simulink model "CrazyFlie"  (R2024a)
settings: Solver=FixedStepAuto  StartTime=0.0  StopTime=8  FixedStep=0.002  RelTol=1e-3
model workspace (MAT data in the model file):
  Bias = 0
  Cd = 7.9379e-12
  ControllerType = 1
  Ct = 3.1582e-10
  Ixx = 1.395e-05
  Iyy = 1.436e-05
  Izz = 2.173e-05
  SampleTime = 0.01
  Ts = 100
  d = 0.06761
  density = 5e-06
undefined symbols (not defined in the file): deg, I, I_inv, k_q, k_t, rad, s
libraries: dspindex x14, simulink_extras x11, aerolibconvert2 x7, uavsim3dlib x3, aerolibutil x2, sharedutil x2, sharedtransform x2, matrix_library x1, sim3dlib x1, uavutilslib x1
settings Model: SnapshotInterval=1  Creator=Guy  LastModifiedBy=User
settings OptimizationCC: ReuseModelBlockBuffer=off
settings ModelReferenceCC: EnableRefExpFcnMdlSchedulingChecks=on
settings RTWCC: GPUComputeCapability=3.5

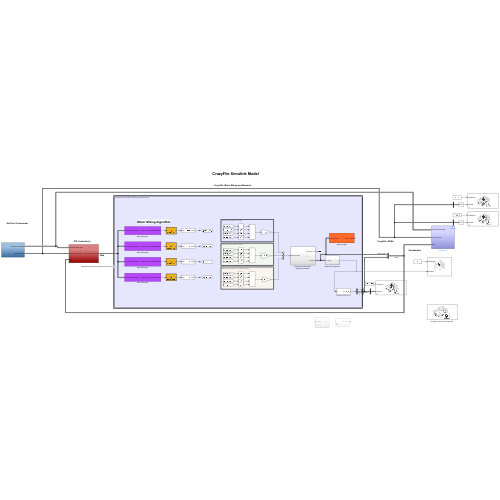
[thumbnail: Simulink's stored preview of the top-level diagram]
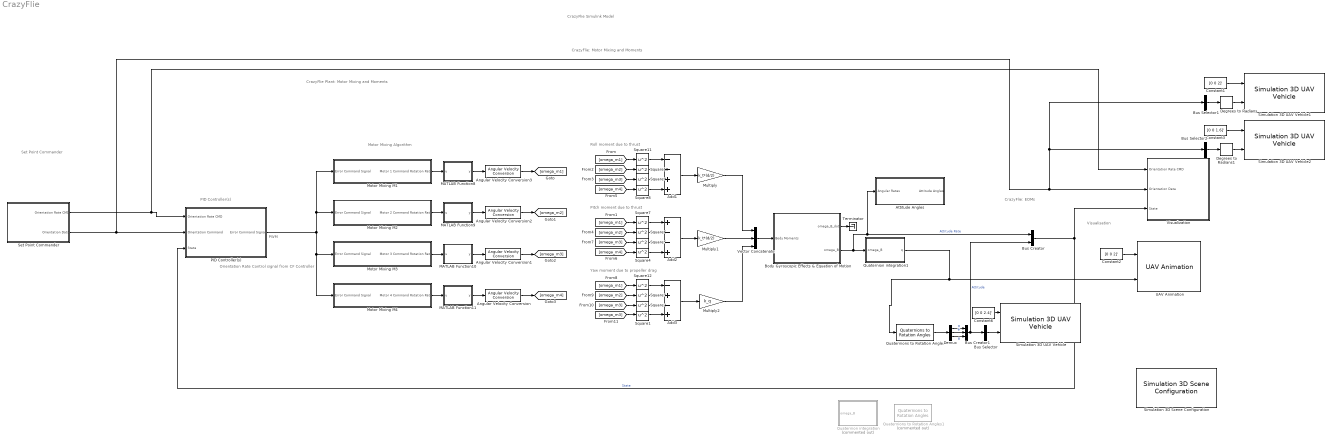
== system CrazyFlie ==
  note: CrazyFlie Plant: Motor Mixing and Moments
  note: PWM
  note: Visualisation
  note: CrazyFlie: EOMs
  note: CrazyFlie: Motor Mixing and Moments
  note: PID Controller(s)
  note: Set Point Commander
  note: CrazyFlie Simulink Model
  note: Orientation Rate Control signal from CF Controller
  note: Motor Mixing Algorithm
  note: Pitch moment due to thrust
  note: Yaw moment due to propeller drag
  note: Roll moment due to thrust
  Add1 : Sum  Inputs=--++
  Add2 : Sum  Inputs=+--+
  Add3 : Sum  Inputs=-+-+
  Angular Velocity Conversion{,1..3} (4 alike) : aerolibconvert2/Angular Velocity Conversion  IU=rpm  OU=rad/s
  Attitude Angles : Subsystem
  Body Gyroscopic Effects & Equation of Motion : Subsystem
  Bus Creator : BusCreator  Inputs=2
  Bus Creator1 : BusCreator  Inputs=3
  Bus Selector : BusSelector  OutputSignals=ψ,Φ,θ  OutputAsBus=on
  Bus Selector1 : BusSelector  OutputSignals=EstimateYaw,EstimatePitch,EstimateRoll  OutputAsBus=on
  Bus Selector2 : BusSelector  OutputSignals=Yaw,Pitch,Roll  OutputAsBus=on
  Constant1 : Constant  Value=[0 0 2]'
  Constant2 : Constant  Value=[0 0 2]'
  Constant3 : Constant  Value=[0 0 1.6]'
  Constant6 : Constant  Value=[0 0 2.4]'
  Degrees to Radians : simulink_extras/Transformations/Degrees to Radians
  Degrees to Radians1 : simulink_extras/Transformations/Degrees to Radians
  Demux : Demux  Outputs=3
  MATLAB Function10 : MATLAB Function  TreatAsAtomicUnit=on
  MATLAB Function11 : MATLAB Function  TreatAsAtomicUnit=on
  MATLAB Function8 : MATLAB Function  TreatAsAtomicUnit=on
  MATLAB Function9 : MATLAB Function  TreatAsAtomicUnit=on
  Motor Mixing M1 : Subsystem
  Motor Mixing M2 : Subsystem
  Motor Mixing M3 : Subsystem
  Motor Mixing M4 : Subsystem
  Multiply : Gain  Gain=k_t*(d/2)
  Multiply1 : Gain  Gain=k_t*(d/2)
  Multiply2 : Gain  Gain=k_q
  PID Controller(s) : Subsystem
  Quaternion integration : Subsystem  Commented=on
  Quaternion integration1 : Subsystem
  Quaternions to Rotation Angles : sharedtransform/Quaternions to Rotation Angles  rotationOrder=ZYX  aMode=aMode
  Quaternions to Rotation Angles1 : sharedtransform/Quaternions to Rotation Angles  Commented=on  rotationOrder=ZYX  aMode=aMode
  Set Point Commander : Subsystem  Tag=Signal Editor
  Simulation 3D Scene Configuration : sim3dlib/Simulation 3D Scene Configuration  Priority=0  ProjectFormat=Default Scenes  SceneDesc=US city block  ProjectName=C:\Program Files\MATLAB\R2024a\toolbox\shared\sim3d_projects\automotive_project_windows\UE\WindowsNoEditor\VehicleSimulation.exe  ScenePath=/Game/Maps/USCityBlock  EnableOpenDRIVE=off  vehTagList={'Custom';'Scene Origin';'SimulinkVehicle1';'SimulinkVehicle2';'SimulinkVehicle3'}  vehTag=Custom  FreeCameraInitialTranslation=[-1.8, 0, 2.6]  FreeCameraDefaultInitialTranslation=[-6, 0, 2]  FreeCameraInitialRotation=[0, -10, 0]  FreeCameraDefaultInitialRotation=[0, -15, 0]  OpVisEn=off  Ts=0.03  EnableWindow=on  EnableRemoteAccess=off  EnableWeather=off  SunAzimuth=90  SunAltitude=40.0  EnableGeospatialSun=off  Latitude=0  Longitude=0  Date=2023-01-01  Time=10:30:00  GeoTimeZone=-5.0  SunDaylightSaving=off  wind=1  clouds=10  EnableVolumetricClouds=off  CloudCoverage=0  CloudAltitude=6  fog=0  rain=0  RaindropsEffect=off  SnowDensity=0  EnableGeospatial=off  UseTrueOrigin=off  OriginHeight=200  OriginLatitude=40.744652  OriginLongitude=-73.988864  MapStyle=Aerial  AdditionalAssetIDs=[]  UseAdvancedSunSky=off  SolarTime=11  TimeZone=-5  Day=21  Month=9  Year=2022  UseDaylightSavingTime=on  DSTStartDay=10  DSTStartMonth=3  DSTEndDay=3  DSTEndMonth=11  DSTSwitchHour=2  sensorTag=MainCamera1  sensorId=1  sensorName=MainCamera1  mountLoc=Origin  offsetFlag=off  tmountOffset=[0, 0, 0]  rmountOffset=[0, 0, 0]  HorizontalResolution=1280  VerticalResolution=720  HorizontalFOV=60  mountPoint=[0 0 0]  mountOrientation=[0 0 0]  aMode=4  ID=1  GeoTrigger=Inactive
      settings: LibrarySourceBlock=uavsim3dlib/Simulation 3D Scene Configuration
  Simulation 3D UAV Vehicle : uavsim3dlib/Simulation 3D UAV Vehicle  Priority=-1  Mesh=Quadrotor  MeshPath=/MathWorksUAVContent/UAVs/HexaRotorUAV/HexaRotor.HexaRotor  Color=Black  ActorName=SimulinkVehicle1  UseGlobalFrame=off  InitialTranslation=[0 0 2.4]  InitialRotation=[0 0 0]  InitialTranslationGlobal=[0 0 0]  InitialGeoOrigin=[0 0 0]  InitialRotationGlobal=[0 0 0]  SampleTime=-1  ActorType=SimulinkVehicle  ID=1  aMode=4  ActorTag=SimulinkVehicle1
  Simulation 3D UAV Vehicle1 : uavsim3dlib/Simulation 3D UAV Vehicle  Priority=-1  Mesh=Quadrotor  MeshPath=/MathWorksUAVContent/UAVs/HexaRotorUAV/HexaRotor.HexaRotor  Color=Black  ActorName=SimulinkVehicle2  UseGlobalFrame=off  InitialTranslation=[0 0 2]  InitialRotation=[0 0 0]  InitialTranslationGlobal=[0 0 0]  InitialGeoOrigin=[0 0 0]  InitialRotationGlobal=[0 0 0]  SampleTime=-1  ActorType=SimulinkVehicle  ID=2  aMode=4  ActorTag=SimulinkVehicle2
  Simulation 3D UAV Vehicle2 : uavsim3dlib/Simulation 3D UAV Vehicle  Priority=-1  Mesh=Quadrotor  MeshPath=/MathWorksUAVContent/UAVs/HexaRotorUAV/HexaRotor.HexaRotor  Color=Black  ActorName=SimulinkVehicle3  UseGlobalFrame=off  InitialTranslation=[0 0 1.6]  InitialRotation=[0 0 0]  InitialTranslationGlobal=[0 0 0]  InitialGeoOrigin=[0 0 0]  InitialRotationGlobal=[0 0 0]  SampleTime=-1  ActorType=SimulinkVehicle  ID=3  aMode=4  ActorTag=SimulinkVehicle3
  Square{1..12} (12 alike) : Math  Operator=square
  Terminator : Terminator
  UAV Animation : uavutilslib/UAV Animation  UAVType=Multirotor  UAVSize=1  InertialZDirection=Up  SampleTime=-1
  Vector Concatenate : Concatenate  NumInputs=3
  Visualization : Subsystem
  wires:
  Set Point Commander/1(Orientation Rate CMD) -> PID Controller(s)/1(Orientation Rate CMD), Visualization/1(Orientation Rate CMD)
  Bus Creator/1 -> PID Controller(s)/3(State), Visualization/3(State)  "State"
  PID Controller(s)/1(Error Command Signal) -> Motor Mixing M1/1(Error Command Signal), Motor Mixing M2/1(Error Command Signal), Motor Mixing M4/1(Error Command Signal), Motor Mixing M3/1(Error Command Signal)
  Motor Mixing M4/1(Motor 4 Command Rotation Rate) -> MATLAB Function11/1(u)
  Motor Mixing M3/1(Motor 3 Command Rotation Rate) -> MATLAB Function10/1(u)
  Motor Mixing M2/1(Motor 2 Command Rotation Rate) -> MATLAB Function9/1(u)
  Motor Mixing M1/1(Motor 1 Command Rotation Rate) -> MATLAB Function8/1(u)
  MATLAB Function8/1(y) -> Angular Velocity Conversion3/1
  MATLAB Function9/1(y) -> Angular Velocity Conversion2/1
  MATLAB Function10/1(y) -> Angular Velocity Conversion1/1
  MATLAB Function11/1(y) -> Angular Velocity Conversion/1
  Angular Velocity Conversion3/1 -> [omega_m1]
  Angular Velocity Conversion2/1 -> [omega_m2]
  Angular Velocity Conversion1/1 -> [omega_m3]
  Angular Velocity Conversion/1 -> [omega_m4]
  Multiply2/1 -> Vector Concatenate/3
  [omega_m1] -> Square7/1
  Multiply/1 -> Vector Concatenate/1
  Vector Concatenate/1 -> Body Gyroscopic Effects & Equation of Motion/1(Body Moments)
  Square11/1 -> Add1/1
  [omega_m3] -> Square9/1
  Square2/1 -> Add3/3
  Square6/1 -> Add2/2
  Multiply1/1 -> Vector Concatenate/2
  [omega_m3] -> Square5/1
  [omega_m4] -> Square8/1
  [omega_m4] -> Square4/1
  Square5/1 -> Add2/3
  Add2/1 -> Multiply1/1
  Square12/1 -> Add3/1
  Square9/1 -> Add1/3
  Add3/1 -> Multiply2/1
  [omega_m3] -> Square2/1
  Square10/1 -> Add1/2
  Add1/1 -> Multiply/1
  Square8/1 -> Add1/4
  [omega_m1] -> Square11/1
  Square7/1 -> Add2/1
  [omega_m2] -> Square6/1
  [omega_m1] -> Square12/1
  [omega_m2] -> Square3/1
  [omega_m2] -> Square10/1
  Square3/1 -> Add3/2
  Square4/1 -> Add2/4
  Body Gyroscopic Effects & Equation of Motion/1(omega_B_dot) -> Terminator/1
  Body Gyroscopic Effects & Equation of Motion/2(omega_B) -> Quaternion integration1/1(omega_B), Attitude Angles/1(Angular Rates), Bus Creator/1  "Attitude Rate"
  Constant6/1 -> Simulation 3D UAV Vehicle/1
  [omega_m3] -> Square1/1
  Square1/1 -> Add3/4
  Set Point Commander/2(Orientation Data) -> PID Controller(s)/2(Orientation Command), Bus Selector1/1, Bus Selector2/1, Visualization/2(Orientation Data)
  Constant1/1 -> Simulation 3D UAV Vehicle1/1
  Bus Selector1/1 -> Degrees to Radians/1
  Degrees to Radians/1 -> Simulation 3D UAV Vehicle1/2
  Quaternion integration1/1(q) -> UAV Animation/2, Quaternions to Rotation Angles/1
  Constant2/1 -> UAV Animation/1
  Bus Selector/1 -> Simulation 3D UAV Vehicle/2
  Degrees to Radians1/1 -> Simulation 3D UAV Vehicle2/2
  Bus Selector2/1 -> Degrees to Radians1/1
  Constant3/1 -> Simulation 3D UAV Vehicle2/1
  Demux/1 -> Bus Creator1/1  "ψ"
  Demux/2 -> Bus Creator1/2  "Φ"
  Demux/3 -> Bus Creator1/3  "θ"
  Bus Creator1/1 -> Bus Creator/2, Bus Selector/1  "Attitude"
  Quaternions to Rotation Angles/1 -> Demux/1

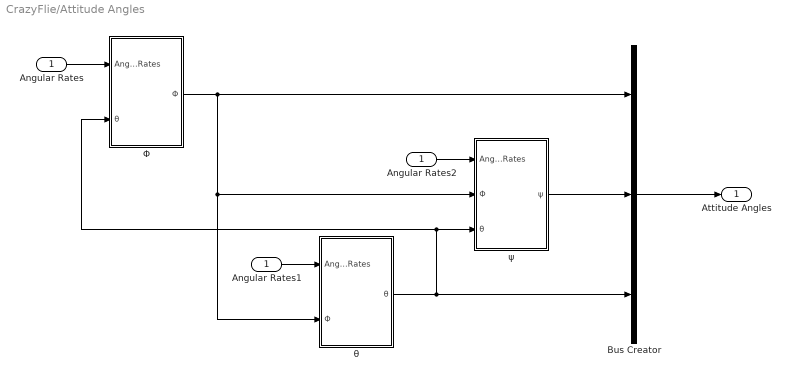
== system CrazyFlie/Attitude Angles ==
  Angular Rates : Inport
  Angular Rates1 : InportShadow
  Angular Rates2 : InportShadow
  Bus Creator : BusCreator  Inputs=3
  Φ : Subsystem
  θ : Subsystem
  ψ : Subsystem
  Attitude Angles : Outport
  wires:
  Angular Rates/1 -> Φ/1(Angular Rates)
  Angular Rates1/1 -> θ/1(Angular Rates)
  Angular Rates2/1 -> ψ/1(Angular Rates)
  θ/1(θ) -> Bus Creator/3, Φ/2(θ), ψ/3(θ)
  Φ/1(Φ) -> θ/2(Φ), ψ/2(Φ), Bus Creator/1
  ψ/1(ψ) -> Bus Creator/2
  Bus Creator/1 -> Attitude Angles/1

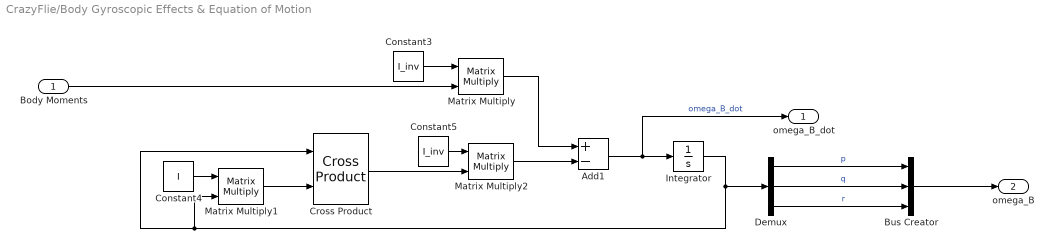
== system CrazyFlie/Body Gyroscopic Effects & Equation of Motion ==
  Body Moments : Inport
  Add1 : Sum  Inputs=+-
  Bus Creator : BusCreator  Inputs=3
  Constant3 : Constant  Value=I_inv
  Constant4 : Constant  Value=I
  Constant5 : Constant  Value=I_inv
  Cross Product : matrix_library/Cross Product
  Demux : Demux  Outputs=3
  Integrator : Integrator
  Matrix Multiply : Product  Multiplication=Matrix(*)
  Matrix Multiply1 : Product  Multiplication=Matrix(*)
  Matrix Multiply2 : Product  Multiplication=Matrix(*)
  omega_B_dot : Outport
  omega_B : Outport  Port=2
  wires:
  Constant4/1 -> Matrix Multiply1/1
  Add1/1 -> omega_B_dot/1, Integrator/1  "omega_B_dot"
  Matrix Multiply2/1 -> Add1/2
  Matrix Multiply1/1 -> Cross Product/2
  Constant3/1 -> Matrix Multiply/1
  Matrix Multiply/1 -> Add1/1
  Cross Product/1 -> Matrix Multiply2/2
  Integrator/1 -> Matrix Multiply1/2, Cross Product/1, Demux/1
  Constant5/1 -> Matrix Multiply2/1
  Body Moments/1 -> Matrix Multiply/2
  Demux/1 -> Bus Creator/1  "p"
  Demux/2 -> Bus Creator/2  "q"
  Demux/3 -> Bus Creator/3  "r"
  Bus Creator/1 -> omega_B/1

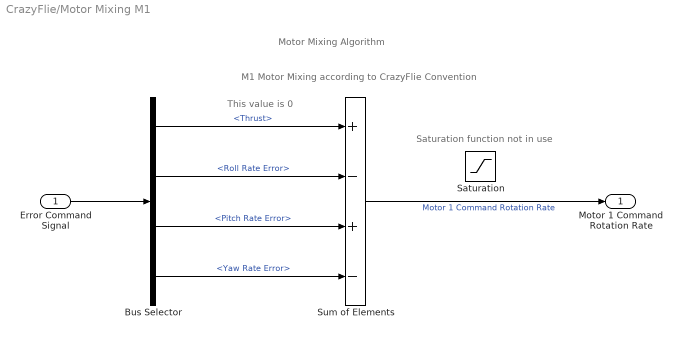
== system CrazyFlie/Motor Mixing M1 ==
  note: Motor Mixing Algorithm
  note: M1 Motor Mixing according to CrazyFlie Convention
  note: This value is 0
  note: Saturation function not in use
  Error Command Signal : Inport
  Bus Selector : BusSelector  OutputSignals=Thrust,Roll Rate Error,Pitch Rate Error,Yaw Rate Error
  Saturation : Saturate
  Sum of Elements : Sum  Inputs=+-+-
  Motor 1 Command Rotation Rate : Outport
  wires:
  Error Command Signal/1 -> Bus Selector/1
  Sum of Elements/1 -> Motor 1 Command Rotation Rate/1  "Motor 1 Command Rotation Rate"
  Bus Selector/3 -> Sum of Elements/3  "<Pitch Rate Error>"
  Bus Selector/4 -> Sum of Elements/4  "<Yaw Rate Error>"
  Bus Selector/2 -> Sum of Elements/2  "<Roll Rate Error>"
  Bus Selector/1 -> Sum of Elements/1  "<Thrust>"

== system CrazyFlie/Motor Mixing M2 ==
  Error Command Signal : Inport
  Bus Selector1 : BusSelector  OutputSignals=Thrust,Roll Rate Error,Pitch Rate Error,Yaw Rate Error
  Sum of Elements1 : Sum  Inputs=+--+
  Motor 2 Command Rotation Rate : Outport
  wires:
  Bus Selector1/4 -> Sum of Elements1/4  "<Yaw Rate Error>"
  Error Command Signal/1 -> Bus Selector1/1
  Bus Selector1/3 -> Sum of Elements1/3  "<Pitch Rate Error>"
  Bus Selector1/1 -> Sum of Elements1/1  "<Thrust>"
  Bus Selector1/2 -> Sum of Elements1/2  "<Roll Rate Error>"
  Sum of Elements1/1 -> Motor 2 Command Rotation Rate/1  "Motor 2 Command Rotation Rate"

== system CrazyFlie/Motor Mixing M3 ==
  Error Command Signal : Inport
  Bus Selector2 : BusSelector  OutputSignals=Thrust,Roll Rate Error,Pitch Rate Error,Yaw Rate Error
  Sum of Elements2 : Sum  Inputs=++--
  Motor 3 Command Rotation Rate : Outport
  wires:
  Bus Selector2/2 -> Sum of Elements2/2  "<Roll Rate Error>"
  Bus Selector2/1 -> Sum of Elements2/1  "<Thrust>"
  Error Command Signal/1 -> Bus Selector2/1
  Bus Selector2/4 -> Sum of Elements2/4  "<Yaw Rate Error>"
  Bus Selector2/3 -> Sum of Elements2/3  "<Pitch Rate Error>"
  Sum of Elements2/1 -> Motor 3 Command Rotation Rate/1  "Motor 3 Command Rotation Rate"

== system CrazyFlie/Motor Mixing M4 ==
  Error Command Signal : Inport
  Bus Selector3 : BusSelector  OutputSignals=Thrust,Roll Rate Error,Pitch Rate Error,Yaw Rate Error
  Sum of Elements3 : Sum  Inputs=++-+
  Motor 4 Command Rotation Rate : Outport
  wires:
  Bus Selector3/4 -> Sum of Elements3/4  "<Yaw Rate Error>"
  Bus Selector3/2 -> Sum of Elements3/2  "<Roll Rate Error>"
  Sum of Elements3/1 -> Motor 4 Command Rotation Rate/1  "Motor 4 Command Rotation Rate"
  Bus Selector3/1 -> Sum of Elements3/1  "<Thrust>"
  Bus Selector3/3 -> Sum of Elements3/3  "<Pitch Rate Error>"
  Error Command Signal/1 -> Bus Selector3/1

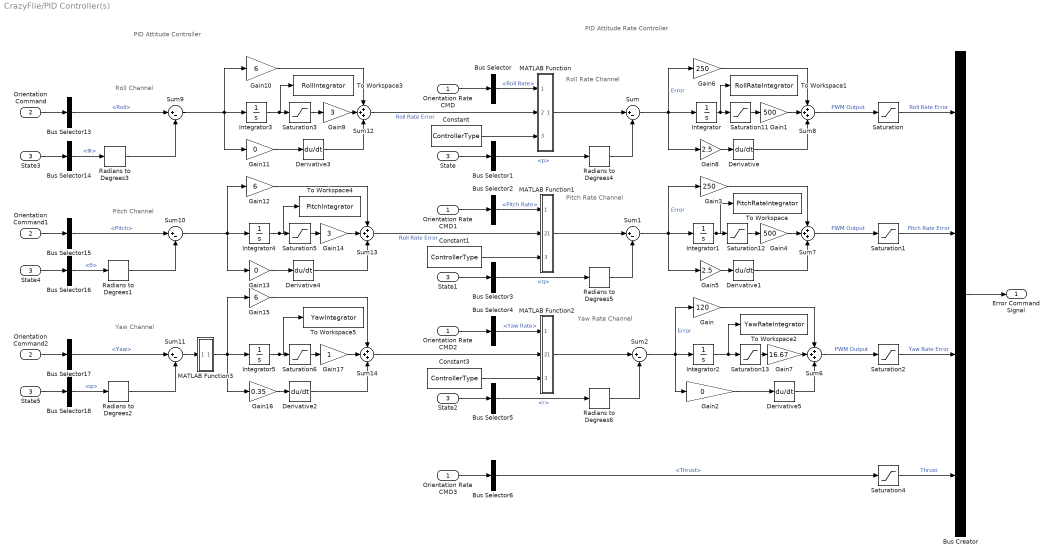
== system CrazyFlie/PID Controller(s) ==
  note: Roll Channel
  note: PID Attitude Controller
  note: PID Attitude Rate Controller
  note: Pitch Channel
  note: Yaw Channel
  note: Roll Rate Channel
  note: Pitch Rate Channel
  note: Yaw Rate Channel
  Orientation Rate CMD : Inport
  Orientation Command : Inport  Port=2
  State : Inport  Port=3
  Bus Creator : BusCreator  Inputs=4
  Bus Selector : BusSelector  OutputSignals=Roll Rate
  Bus Selector1 : BusSelector  OutputSignals=Attitude Rate.p
  Bus Selector13 : BusSelector  OutputSignals=Roll
  Bus Selector14 : BusSelector  OutputSignals=Attitude.Φ
  Bus Selector15 : BusSelector  OutputSignals=Pitch
  Bus Selector16 : BusSelector  OutputSignals=Attitude.θ
  Bus Selector17 : BusSelector  OutputSignals=Yaw
  Bus Selector18 : BusSelector  OutputSignals=Attitude.ψ
  Bus Selector2 : BusSelector  OutputSignals=Pitch Rate
  Bus Selector3 : BusSelector  OutputSignals=Attitude Rate.q
  Bus Selector4 : BusSelector  OutputSignals=Yaw Rate
  Bus Selector5 : BusSelector  OutputSignals=Attitude Rate.r
  Bus Selector6 : BusSelector  OutputSignals=Thrust
  Constant : Constant  Value=ControllerType
  Constant1 : Constant  Value=ControllerType
  Constant3 : Constant  Value=ControllerType
  Derivative{,1..5} (6 alike) : Derivative
  Gain : Gain  Gain=120
  Gain1 : Gain  Gain=500
  Gain10 : Gain  Gain=6
  Gain11 : Gain  Gain=0
  Gain12 : Gain  Gain=6
  Gain13 : Gain  Gain=0
  Gain14 : Gain  Gain=3
  Gain15 : Gain  Gain=6
  Gain16 : Gain  Gain=0.35
  Gain17 : Gain
  Gain2 : Gain  Gain=0
  Gain3 : Gain  Gain=250
  Gain4 : Gain  Gain=500
  Gain5 : Gain  Gain=2.5
  Gain6 : Gain  Gain=250
  Gain7 : Gain  Gain=16.67
  Gain8 : Gain  Gain=2.5
  Gain9 : Gain  Gain=3
  Integrator : Integrator  InitialCondition=-61  UpperSaturationLimit=33.33  LowerSaturationLimit=-33.33
  Integrator1 : Integrator  InitialCondition=61
  Integrator2 : Integrator
  Integrator3 : Integrator
  Integrator4 : Integrator
  Integrator5 : Integrator  InitialCondition=0.47
  MATLAB Function : MATLAB Function  TreatAsAtomicUnit=on
  MATLAB Function1 : MATLAB Function  TreatAsAtomicUnit=on
  MATLAB Function2 : MATLAB Function  TreatAsAtomicUnit=on
  MATLAB Function3 : MATLAB Function  TreatAsAtomicUnit=on
  Orientation Command1 : InportShadow  Port=2
  Orientation Command2 : InportShadow  Port=2
  Orientation Rate CMD1 : InportShadow
  Orientation Rate CMD2 : InportShadow
  Orientation Rate CMD3 : InportShadow
  Radians to Degrees{1..6} (6 alike) : simulink_extras/Transformations/Radians to Degrees
  Saturation : Saturate  UpperLimit=2767  LowerLimit=-62768  LinearizeAsGain=off  ZeroCross=off
  Saturation1 : Saturate  UpperLimit=62767  LowerLimit=-32768  LinearizeAsGain=off  ZeroCross=off
  Saturation{3,5..6,11..13} (6 alike) : Saturate  UpperLimit=inf  LowerLimit=-inf
  Saturation2 : Saturate  UpperLimit=32767  LowerLimit=-32768  LinearizeAsGain=off  ZeroCross=off
  Saturation4 : Saturate  UpperLimit=0  LowerLimit=0  LinearizeAsGain=off  ZeroCross=off
  State{1..5} (5 alike) : InportShadow  Port=3
  Sum{,1..2,9..11} (6 alike) : Sum  Inputs=|+-
  Sum{6..8,12..14} (6 alike) : Sum  Inputs=+++
  To Workspace : ToWorkspace  VariableName=PitchRateIntegrator  SaveFormat=Timeseries  SampleTime=0.01
  To Workspace1 : ToWorkspace  VariableName=RollRateIntegrator  SaveFormat=Timeseries  SampleTime=0.01
  To Workspace2 : ToWorkspace  VariableName=YawRateIntegrator  SaveFormat=Timeseries  SampleTime=-1
  To Workspace3 : ToWorkspace  VariableName=RollIntegrator  SaveFormat=Timeseries  SampleTime=0.01
  To Workspace4 : ToWorkspace  VariableName=PitchIntegrator  SaveFormat=Timeseries  SampleTime=0.01
  To Workspace5 : ToWorkspace  VariableName=YawIntegrator  SaveFormat=Timeseries  SampleTime=0.01
  Error Command Signal : Outport
  wires:
  Orientation Rate CMD/1 -> Bus Selector/1
  State/1 -> Bus Selector1/1
  Bus Selector1/1 -> Radians to Degrees4/1  "<p>"
  Bus Selector3/1 -> Radians to Degrees5/1  "<q>"
  Orientation Rate CMD1/1 -> Bus Selector2/1
  State1/1 -> Bus Selector3/1
  Bus Selector5/1 -> Radians to Degrees6/1  "<r>"
  Orientation Rate CMD2/1 -> Bus Selector4/1
  State2/1 -> Bus Selector5/1
  Bus Creator/1 -> Error Command Signal/1
  Orientation Rate CMD3/1 -> Bus Selector6/1
  Bus Selector6/1 -> Saturation4/1  "<Thrust>"
  Gain/1 -> Sum6/1
  Sum6/1 -> Saturation2/1  "PWM Output"
  Gain3/1 -> Sum7/1
  Sum7/1 -> Saturation1/1  "PWM Output"
  Sum1/1 -> Integrator1/1, Gain5/1, Gain3/1  "Error"
  Gain6/1 -> Sum8/1
  Gain8/1 -> Derivative/1
  Sum/1 -> Integrator/1, Gain8/1, Gain6/1  "Error"
  Sum8/1 -> Saturation/1  "PWM Output"
  Saturation/1 -> Bus Creator/1  "Roll Rate Error"
  Saturation1/1 -> Bus Creator/2  "Pitch Rate Error"
  Saturation2/1 -> Bus Creator/3  "Yaw Rate Error"
  Gain5/1 -> Derivative1/1
  Derivative1/1 -> Sum7/3
  Derivative/1 -> Sum8/3
  Gain1/1 -> Sum8/2
  Gain4/1 -> Sum7/2
  Sum2/1 -> Integrator2/1, Gain/1, Gain2/1  "Error"
  Gain7/1 -> Sum6/2
  Integrator/1 -> Saturation11/1, To Workspace1/1
  Integrator1/1 -> To Workspace/1, Saturation12/1
  Integrator2/1 -> Saturation13/1, To Workspace2/1
  Saturation4/1 -> Bus Creator/4  "Thrust"
  Orientation Command/1 -> Bus Selector13/1
  State3/1 -> Bus Selector14/1
  Orientation Command1/1 -> Bus Selector15/1
  State4/1 -> Bus Selector16/1
  Orientation Command2/1 -> Bus Selector17/1
  State5/1 -> Bus Selector18/1
  Bus Selector14/1 -> Radians to Degrees3/1  "<Φ>"
  Bus Selector16/1 -> Radians to Degrees1/1  "<θ>"
  Bus Selector18/1 -> Radians to Degrees2/1  "<ψ>"
  Sum9/1 -> Integrator3/1, Gain11/1, Gain10/1
  Derivative3/1 -> Sum12/3
  Gain11/1 -> Derivative3/1
  Gain10/1 -> Sum12/1
  Gain9/1 -> Sum12/2
  Sum10/1 -> Gain13/1, Integrator4/1, Gain12/1
  Gain12/1 -> Sum13/1
  Gain14/1 -> Sum13/2
  Derivative4/1 -> Sum13/3
  Gain13/1 -> Derivative4/1
  Gain15/1 -> Sum14/1
  Gain17/1 -> Sum14/2
  Derivative2/1 -> Sum14/3
  Gain16/1 -> Derivative2/1
  Saturation11/1 -> Gain1/1
  Saturation12/1 -> Gain4/1
  Saturation13/1 -> Gain7/1
  Gain2/1 -> Derivative5/1
  Integrator3/1 -> Saturation3/1, To Workspace3/1
  Integrator4/1 -> To Workspace4/1, Saturation5/1
  Integrator5/1 -> To Workspace5/1, Saturation6/1
  Saturation3/1 -> Gain9/1
  Saturation5/1 -> Gain14/1
  Saturation6/1 -> Gain17/1
  Radians to Degrees3/1 -> Sum9/2
  Radians to Degrees1/1 -> Sum10/2
  Radians to Degrees2/1 -> Sum11/2
  MATLAB Function3/1(y) -> Integrator5/1, Gain16/1, Gain15/1
  Sum11/1 -> MATLAB Function3/1(YawError)
  Derivative5/1 -> Sum6/3
  Radians to Degrees4/1 -> Sum/2
  Radians to Degrees5/1 -> Sum1/2
  Radians to Degrees6/1 -> Sum2/2
  Constant/1 -> MATLAB Function/3(type)
  Constant1/1 -> MATLAB Function1/3(type)
  Constant3/1 -> MATLAB Function2/3(type)
  Sum12/1 -> MATLAB Function/2(Angle)  "Roll Rate Error"
  Sum13/1 -> MATLAB Function1/2(Angle)  "Roll Rate Error"
  Sum14/1 -> MATLAB Function2/2(Angle)
  Bus Selector17/1 -> Sum11/1  "<Yaw>"
  Bus Selector15/1 -> Sum10/1  "<Pitch>"
  Bus Selector13/1 -> Sum9/1  "<Roll>"
  MATLAB Function/1(y) -> Sum/1
  MATLAB Function1/1(y) -> Sum1/1
  Bus Selector2/1 -> MATLAB Function1/1(Rate)  "<Pitch Rate>"
  Bus Selector/1 -> MATLAB Function/1(Rate)  "<Roll Rate>"
  MATLAB Function2/1(y) -> Sum2/1
  Bus Selector4/1 -> MATLAB Function2/1(Rate)  "<Yaw Rate>"

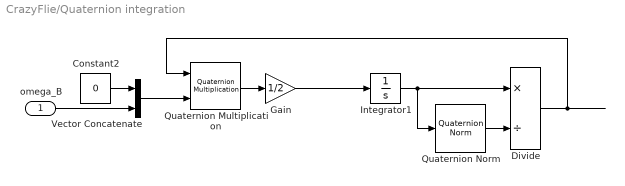
== system CrazyFlie/Quaternion integration ==
  omega_B : Inport
  Constant2 : Constant  Value=0
  Divide : Product  Inputs=*/
  Gain : Gain  Gain=1/2
  Integrator1 : Integrator  InitialCondition=[1 0 0 0]'
  Quaternion Multiplication : aerolibutil/Quaternion Multiplication
  Quaternion Norm : sharedutil/Quaternion Norm  aMode=aMode
      settings: LibrarySourceBlock=|
      | aerolibutil/Quaternion
      | Norm
  Vector Concatenate : Concatenate
  wires:
  Divide/1 -> Quaternion Multiplication/1
  Integrator1/1 -> Quaternion Norm/1, Divide/1
  Constant2/1 -> Vector Concatenate/1
  Quaternion Multiplication/1 -> Gain/1
  Vector Concatenate/1 -> Quaternion Multiplication/2
  Gain/1 -> Integrator1/1
  Quaternion Norm/1 -> Divide/2
  omega_B/1 -> Vector Concatenate/2

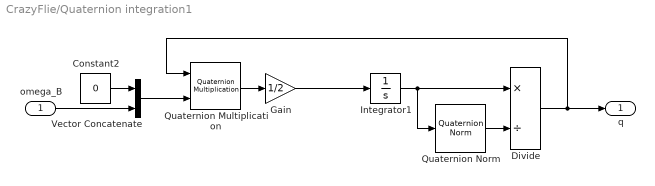
== system CrazyFlie/Quaternion integration1 ==
  omega_B : Inport
  Constant2 : Constant  Value=0
  Divide : Product  Inputs=*/
  Gain : Gain  Gain=1/2
  Integrator1 : Integrator  InitialCondition=[1 0 0 0]'
  Quaternion Multiplication : aerolibutil/Quaternion Multiplication
  Quaternion Norm : sharedutil/Quaternion Norm  aMode=aMode
      settings: LibrarySourceBlock=|
      | aerolibutil/Quaternion
      | Norm
  Vector Concatenate : Concatenate
  q : Outport
  wires:
  Divide/1 -> Quaternion Multiplication/1, q/1
  Integrator1/1 -> Quaternion Norm/1, Divide/1
  Constant2/1 -> Vector Concatenate/1
  Quaternion Multiplication/1 -> Gain/1
  Vector Concatenate/1 -> Quaternion Multiplication/2
  Gain/1 -> Integrator1/1
  Quaternion Norm/1 -> Divide/2
  omega_B/1 -> Vector Concatenate/2

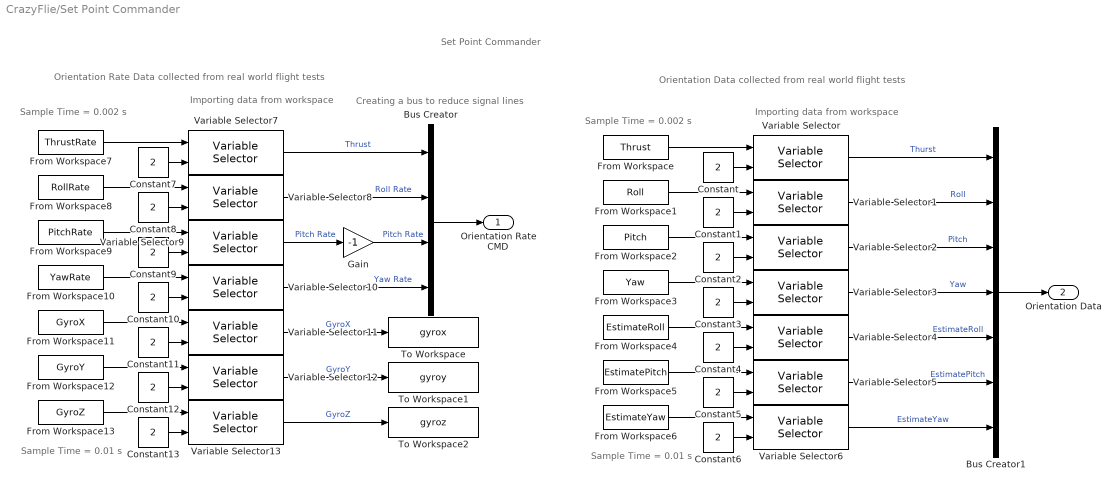
== system CrazyFlie/Set Point Commander ==
  note: Creating a bus to reduce signal lines
  note: Sample Time = 0.002 s
  note: Set Point Commander
  note: Importing data from workspace
  note: Importing data from workspace
  note: Orientation Rate Data collected from real world flight tests
  note: Orientation Data collected from real world flight tests
  note: Sample Time = 0.002 s
  note: Sample Time = 0.01 s
  note: Sample Time = 0.01 s
  Bus Creator : BusCreator  Inputs=4
  Bus Creator1 : BusCreator  Inputs=7
  Constant{,1..13} (14 alike) : Constant  Value=2
  From Workspace : FromWorkspace  VariableName=Thrust  SampleTime=0.002  OutputAfterFinalValue=Holding final value
  From Workspace1 : FromWorkspace  VariableName=Roll  SampleTime=0.002  OutputAfterFinalValue=Setting to zero
  From Workspace10 : FromWorkspace  VariableName=YawRate  SampleTime=0.002  OutputAfterFinalValue=Setting to zero
  From Workspace11 : FromWorkspace  VariableName=GyroX  SampleTime=0.002  OutputAfterFinalValue=Setting to zero
  From Workspace12 : FromWorkspace  VariableName=GyroY  SampleTime=0.002  OutputAfterFinalValue=Setting to zero
  From Workspace13 : FromWorkspace  VariableName=GyroZ  SampleTime=0.002  OutputAfterFinalValue=Setting to zero
  From Workspace2 : FromWorkspace  VariableName=Pitch  SampleTime=0.002  OutputAfterFinalValue=Setting to zero
  From Workspace3 : FromWorkspace  VariableName=Yaw  SampleTime=0.002  OutputAfterFinalValue=Setting to zero
  From Workspace4 : FromWorkspace  VariableName=EstimateRoll  SampleTime=0.002  OutputAfterFinalValue=Setting to zero
  From Workspace5 : FromWorkspace  VariableName=EstimatePitch  SampleTime=0.002  OutputAfterFinalValue=Setting to zero
  From Workspace6 : FromWorkspace  VariableName=EstimateYaw  SampleTime=0.002  OutputAfterFinalValue=Setting to zero
  From Workspace7 : FromWorkspace  VariableName=ThrustRate  SampleTime=0.002  OutputAfterFinalValue=Holding final value
  From Workspace8 : FromWorkspace  VariableName=RollRate  SampleTime=0.002  OutputAfterFinalValue=Holding final value
  From Workspace9 : FromWorkspace  VariableName=PitchRate  SampleTime=0.002  OutputAfterFinalValue=Setting to zero
  Gain : Gain  Gain=-1
  To Workspace : ToWorkspace  VariableName=gyrox  SaveFormat=Timeseries  SampleTime=0.002
  To Workspace1 : ToWorkspace  VariableName=gyroy  SaveFormat=Timeseries  SampleTime=0.002
  To Workspace2 : ToWorkspace  VariableName=gyroz  SaveFormat=Timeseries  SampleTime=0.002
  Variable Selector{,1..13} (14 alike) : dspindex/Variable Selector  NumInputs=1  rowsOrCols=Columns  IdxMode=Variable  Elements=[1 3]  ZerOneIdxMode=One-based  errmode=Clip Index  FillMode=off  FillValues=0
  Orientation Rate CMD : Outport
  Orientation Data : Outport  Port=2
  wires:
  Bus Creator/1 -> Orientation Rate CMD/1
  From Workspace/1 -> Variable Selector/1
  Bus Creator1/1 -> Orientation Data/1
  From Workspace1/1 -> Variable Selector1/1
  From Workspace2/1 -> Variable Selector2/1
  From Workspace5/1 -> Variable Selector5/1
  From Workspace3/1 -> Variable Selector3/1
  From Workspace4/1 -> Variable Selector4/1
  From Workspace6/1 -> Variable Selector6/1
  Variable Selector6/1 -> Bus Creator1/7  "EstimateYaw"
  Variable Selector5/1 -> Bus Creator1/6  "EstimatePitch"
  Variable Selector4/1 -> Bus Creator1/5  "EstimateRoll"
  Variable Selector3/1 -> Bus Creator1/4  "Yaw"
  Variable Selector2/1 -> Bus Creator1/3  "Pitch"
  Variable Selector1/1 -> Bus Creator1/2  "Roll"
  Variable Selector/1 -> Bus Creator1/1  "Thurst"
  Constant1/1 -> Variable Selector1/2
  Constant/1 -> Variable Selector/2
  Constant2/1 -> Variable Selector2/2
  Constant3/1 -> Variable Selector3/2
  Constant4/1 -> Variable Selector4/2
  Constant5/1 -> Variable Selector5/2
  Constant6/1 -> Variable Selector6/2
  Constant13/1 -> Variable Selector13/2
  Constant11/1 -> Variable Selector11/2
  Constant8/1 -> Variable Selector8/2
  Constant12/1 -> Variable Selector12/2
  Constant9/1 -> Variable Selector9/2
  From Workspace8/1 -> Variable Selector8/1
  From Workspace13/1 -> Variable Selector13/1
  From Workspace12/1 -> Variable Selector12/1
  Constant10/1 -> Variable Selector10/2
  From Workspace10/1 -> Variable Selector10/1
  From Workspace9/1 -> Variable Selector9/1
  From Workspace7/1 -> Variable Selector7/1
  Constant7/1 -> Variable Selector7/2
  From Workspace11/1 -> Variable Selector11/1
  Variable Selector7/1 -> Bus Creator/1  "Thrust"
  Variable Selector8/1 -> Bus Creator/2  "Roll Rate"
  Variable Selector9/1 -> Gain/1  "Pitch Rate"
  Variable Selector10/1 -> Bus Creator/4  "Yaw Rate"
  Variable Selector11/1 -> To Workspace/1  "GyroX"
  Variable Selector12/1 -> To Workspace1/1  "GyroY"
  Variable Selector13/1 -> To Workspace2/1  "GyroZ"
  Gain/1 -> Bus Creator/3  "Pitch Rate"

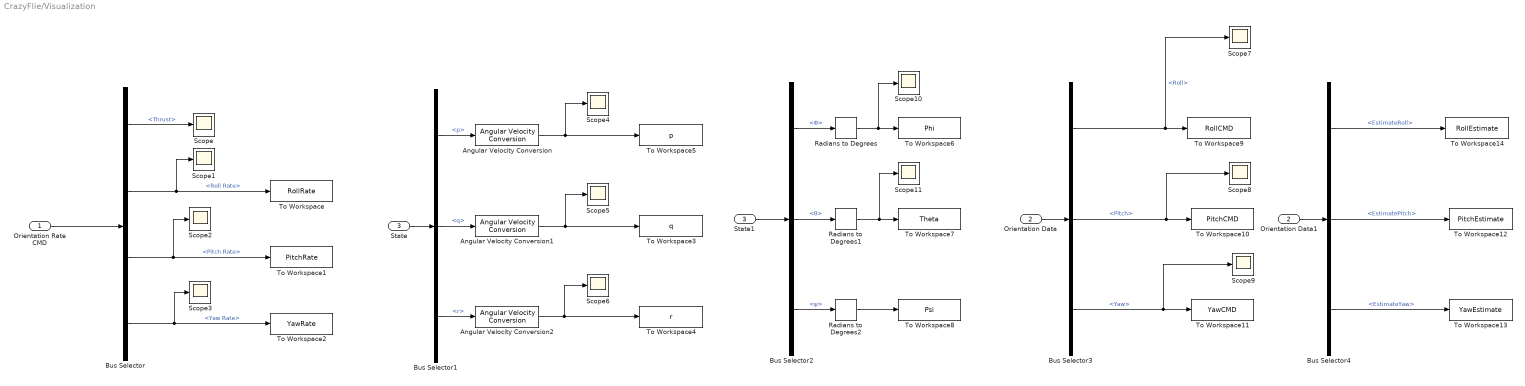
== system CrazyFlie/Visualization ==
  Orientation Rate CMD : Inport
  Orientation Data : Inport  Port=2
  State : Inport  Port=3
  Angular Velocity Conversion : aerolibconvert2/Angular Velocity Conversion  IU=rad/s  OU=deg/s
  Angular Velocity Conversion1 : aerolibconvert2/Angular Velocity Conversion  IU=rad/s  OU=deg/s
  Angular Velocity Conversion2 : aerolibconvert2/Angular Velocity Conversion  IU=rad/s  OU=deg/s
  Bus Selector : BusSelector  OutputSignals=Thrust,Roll Rate,Pitch Rate,Yaw Rate
  Bus Selector1 : BusSelector  OutputSignals=Attitude Rate.p,Attitude Rate.q,Attitude Rate.r
  Bus Selector2 : BusSelector  OutputSignals=Attitude.Φ,Attitude.θ,Attitude.ψ
  Bus Selector3 : BusSelector  OutputSignals=Roll,Pitch,Yaw
  Bus Selector4 : BusSelector  OutputSignals=EstimateRoll,EstimatePitch,EstimateYaw
  Orientation Data1 : InportShadow  Port=2
  Radians to Degrees : simulink_extras/Transformations/Radians to Degrees
  Radians to Degrees1 : simulink_extras/Transformations/Radians to Degrees
  Radians to Degrees2 : simulink_extras/Transformations/Radians to Degrees
  Scope{,1..11} (12 alike) : Scope
  State1 : InportShadow  Port=3
  To Workspace : ToWorkspace  VariableName=RollRate  SaveFormat=Timeseries  SampleTime=0.002
  To Workspace1 : ToWorkspace  VariableName=PitchRate  SaveFormat=Timeseries  SampleTime=0.002
  To Workspace10 : ToWorkspace  VariableName=PitchCMD  SaveFormat=Timeseries  SampleTime=0.002
  To Workspace11 : ToWorkspace  VariableName=YawCMD  SaveFormat=Timeseries  SampleTime=0.002
  To Workspace12 : ToWorkspace  VariableName=PitchEstimate  SaveFormat=Timeseries  SampleTime=0.002
  To Workspace13 : ToWorkspace  VariableName=YawEstimate  SaveFormat=Timeseries  SampleTime=0.002
  To Workspace14 : ToWorkspace  VariableName=RollEstimate  SaveFormat=Timeseries  SampleTime=0.002
  To Workspace2 : ToWorkspace  VariableName=YawRate  SaveFormat=Timeseries  SampleTime=0.002
  To Workspace3 : ToWorkspace  VariableName=q  SaveFormat=Timeseries  SampleTime=0.002
  To Workspace4 : ToWorkspace  VariableName=r  SaveFormat=Timeseries  SampleTime=0.002
  To Workspace5 : ToWorkspace  VariableName=p  SaveFormat=Timeseries  SampleTime=0.002
  To Workspace6 : ToWorkspace  VariableName=Phi  SaveFormat=Timeseries  SampleTime=0.002
  To Workspace7 : ToWorkspace  VariableName=Theta  SaveFormat=Timeseries  SampleTime=0.002
  To Workspace8 : ToWorkspace  VariableName=Psi  SaveFormat=Timeseries  SampleTime=0.002
  To Workspace9 : ToWorkspace  VariableName=RollCMD  SaveFormat=Timeseries  SampleTime=0.002
  wires:
  Orientation Rate CMD/1 -> Bus Selector/1
  Bus Selector/1 -> Scope/1  "<Thrust>"
  Bus Selector/2 -> To Workspace/1, Scope1/1  "<Roll Rate>"
  Bus Selector/3 -> To Workspace1/1, Scope2/1  "<Pitch Rate>"
  Bus Selector/4 -> To Workspace2/1, Scope3/1  "<Yaw Rate>"
  Bus Selector1/2 -> Angular Velocity Conversion1/1  "<q>"
  State/1 -> Bus Selector1/1
  Bus Selector1/3 -> Angular Velocity Conversion2/1  "<r>"
  Bus Selector1/1 -> Angular Velocity Conversion/1  "<p>"
  Angular Velocity Conversion/1 -> To Workspace5/1, Scope4/1
  Angular Velocity Conversion1/1 -> To Workspace3/1, Scope5/1
  Angular Velocity Conversion2/1 -> To Workspace4/1, Scope6/1
  State1/1 -> Bus Selector2/1
  Bus Selector2/3 -> Radians to Degrees2/1  "<ψ>"
  Bus Selector2/2 -> Radians to Degrees1/1  "<θ>"
  Bus Selector2/1 -> Radians to Degrees/1  "<Φ>"
  Bus Selector3/2 -> Scope8/1, To Workspace10/1  "<Pitch>"
  Bus Selector3/3 -> Scope9/1, To Workspace11/1  "<Yaw>"
  Bus Selector3/1 -> Scope7/1, To Workspace9/1  "<Roll>"
  Orientation Data/1 -> Bus Selector3/1
  Bus Selector4/1 -> To Workspace14/1  "<EstimateRoll>"
  Orientation Data1/1 -> Bus Selector4/1
  Bus Selector4/2 -> To Workspace12/1  "<EstimatePitch>"
  Bus Selector4/3 -> To Workspace13/1  "<EstimateYaw>"
  Radians to Degrees/1 -> Scope10/1, To Workspace6/1
  Radians to Degrees1/1 -> Scope11/1, To Workspace7/1
  Radians to Degrees2/1 -> To Workspace8/1

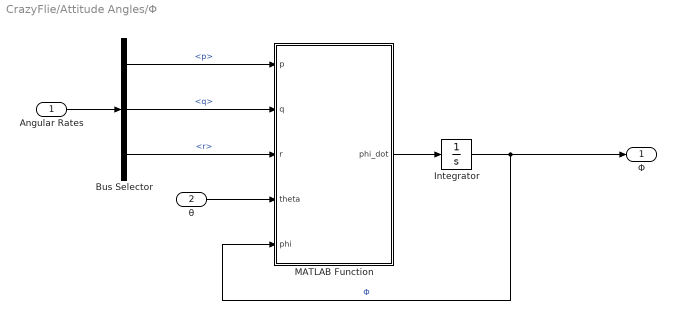
== system CrazyFlie/Attitude Angles/Φ ==
  Angular Rates : Inport
  θ : Inport  Port=2
  Bus Selector : BusSelector  OutputSignals=p,q,r
  Integrator : Integrator
  MATLAB Function : MATLAB Function  TreatAsAtomicUnit=on
  Φ : Outport
  wires:
  Angular Rates/1 -> Bus Selector/1
  θ/1 -> MATLAB Function/4(theta)
  Bus Selector/1 -> MATLAB Function/1(p)  "<p>"
  Bus Selector/2 -> MATLAB Function/2(q)  "<q>"
  Bus Selector/3 -> MATLAB Function/3(r)  "<r>"
  MATLAB Function/1(phi_dot) -> Integrator/1
  Integrator/1 -> Φ/1, MATLAB Function/5(phi)  "Φ"

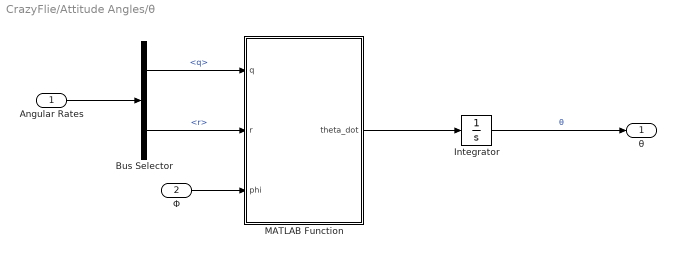
== system CrazyFlie/Attitude Angles/θ ==
  Angular Rates : Inport
  Φ : Inport  Port=2
  Bus Selector : BusSelector  OutputSignals=q,r
  Integrator : Integrator
  MATLAB Function : MATLAB Function  TreatAsAtomicUnit=on
  θ : Outport
  wires:
  Angular Rates/1 -> Bus Selector/1
  Integrator/1 -> θ/1  "θ"
  Bus Selector/1 -> MATLAB Function/1(q)  "<q>"
  Bus Selector/2 -> MATLAB Function/2(r)  "<r>"
  Φ/1 -> MATLAB Function/3(phi)
  MATLAB Function/1(theta_dot) -> Integrator/1

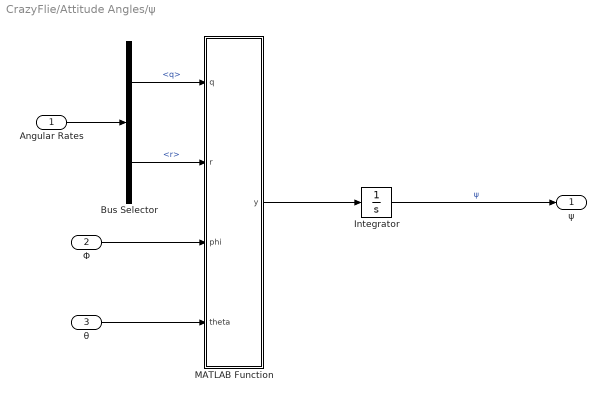
== system CrazyFlie/Attitude Angles/ψ ==
  Angular Rates : Inport
  Φ : Inport  Port=2
  θ : Inport  Port=3
  Bus Selector : BusSelector  OutputSignals=q,r
  Integrator : Integrator
  MATLAB Function : MATLAB Function  TreatAsAtomicUnit=on
  ψ : Outport
  wires:
  Angular Rates/1 -> Bus Selector/1
  Integrator/1 -> ψ/1  "ψ"
  Bus Selector/1 -> MATLAB Function/1(q)  "<q>"
  Bus Selector/2 -> MATLAB Function/2(r)  "<r>"
  Φ/1 -> MATLAB Function/3(phi)
  θ/1 -> MATLAB Function/4(theta)
  MATLAB Function/1(y) -> Integrator/1

== matlab function CrazyFlie/MATLAB Function8 ==
  data: u input; y output
function y = PWMtoRPM(u)

y = u*0.2685+4070.3;

== matlab function CrazyFlie/MATLAB Function9 ==
  data: u input; y output
function y = PWMtoRPM(u)

y = u*0.2685+4070.3;

== matlab function CrazyFlie/MATLAB Function10 ==
  data: u input; y output
function y = PWMtoRPM(u)

y = u*0.2685+4070.3;

== matlab function CrazyFlie/MATLAB Function11 ==
  data: u input; y output
function y = PWMtoRPM(u)

y = u*0.2685+4070.3;

== matlab function CrazyFlie/PID Controller(s)/MATLAB Function3 ==
  data: YawError input; y output
function y = fcn(YawError)
YawError1=YawError;
if YawError>180
    YawError1=YawError-360;
end 
if YawError<-180
    YawError1=YawError+360;
end

y = YawError1;

== matlab function CrazyFlie/PID Controller(s)/MATLAB Function ==
  data: Rate input; Angle input; y output; type input
function y = fcn(Rate,Angle, type)
yy=0;
if type==1
    yy=Angle;
end
if type==2
    yy=Rate;
end

y=yy;

== matlab function CrazyFlie/PID Controller(s)/MATLAB Function1 ==
  data: Rate input; Angle input; y output; type input
function y = fcn(Rate,Angle, type)
yy=0;
if type==1
    yy=Angle;
end
if type==2
    yy=Rate;
end

y=yy;

== matlab function CrazyFlie/PID Controller(s)/MATLAB Function2 ==
  data: Rate input; Angle input; y output; type input
function y = fcn(Rate,Angle,type)
yy=0;
if type==1
    yy=Angle;
end
if type==2
    yy=Rate;
end
y=yy;

== matlab function CrazyFlie/Attitude Angles/Φ/MATLAB Function ==
  data: p input; phi_dot output; q input; r input; theta input; phi input
function phi_dot = fcn(p,q,r,theta,phi)

phi_dot= p+q*sin(phi)*tan(theta)+r*cos(phi)*tan(theta);

== matlab function CrazyFlie/Attitude Angles/θ/MATLAB Function ==
  data: q input; theta_dot output; r input; phi input
function theta_dot = fcn(q,r,phi)

theta_dot = q*cos(phi)-sin(phi)*r;

== matlab function CrazyFlie/Attitude Angles/ψ/MATLAB Function ==
  data: q input; y output; r input; phi input; theta input
function y = fcn(q,r,phi,theta)

y = (q*sin(phi)+r*cos(phi))*sec(theta);
